simulink model "rlObstacleAvoidance"  (R2019b)
settings: Solver=ode23t  StartTime=0.0  StopTime=inf  RelTol=1e-3
InitFcn:
  | close all;
  | clear showPath;
  | lidarNoiseSeeds = randi(intmax,size(scanAngles));
model workspace (MAT data in the model file):
  mapForSim.obsMap = [0 0 0 0 0 0 0 0 0 0 0 0 ... (25000 elements, 200x125)]
  mapForSim.scaleFactor = 25
  mapForSim.simMap = robotics.BinaryOccupancyGrid
  mapForSim.simMap.Grid = [1 1 1 1 1 1 1 1 1 1 1 1 ... (25000 elements, 200x125)]
  mapForSim.simMap.LayerName = "binaryLayer"
  mapForSim.simMap.Index = matlabshared.autonomous.internal.CircularBufferIndex
  mapForSim.simMap.Index.Head = [1 1]
  mapForSim.simMap.Index.Size = [200 125]
  mapForSim.simMap.Index.NewRegions = [0 0 0 0]
  mapForSim.simMap.Index.DropEntireMap = 0
  mapForSim.simMap.Index.DropTwoRegions = [0 0]
  mapForSim.simMap.Buffer = matlabshared.autonomous.internal.CircularBuffer
  mapForSim.simMap.Buffer.ConstVal = 0
  mapForSim.simMap.Buffer.DataType = 'logical'
  mapForSim.simMap.Buffer.Index = matlabshared.autonomous.internal.CircularBufferIndex
  mapForSim.simMap.Buffer.Index.Head = [1 1]
  mapForSim.simMap.Buffer.Index.Size = [200 125]
  mapForSim.simMap.Buffer.Index.NewRegions = [0 0 0 0]
  mapForSim.simMap.Buffer.Index.DropEntireMap = 0
  mapForSim.simMap.Buffer.Index.DropTwoRegions = [0 0]
  mapForSim.simMap.Buffer.Buffer = [1 1 1 1 1 1 1 1 1 1 1 1 ... (25000 elements, 200x125)]
  mapForSim.simMap.DefaultValueInternal = 0
  mapForSim.simMap.HasParent = 0
  mapForSim.simMap.Resolution = 25
  mapForSim.simMap.GridSize = [200 125]
  mapForSim.simMap.GridOriginInLocal = [0 0]
  mapForSim.simMap.LocalOriginInWorld = [0 0]
  mapForSim.simMap.Width = 5
  mapForSim.simMap.Height = 8
  mapForSim.simMap.LocalOriginInWorldInternal = [0 0]
  occGrid = robotics.BinaryOccupancyGrid
  occGrid.Grid = [1 1 1 1 1 1 1 1 1 1 1 1 ... (25000 elements, 200x125)]
  occGrid.LayerName = "binaryLayer"
  occGrid.Index = matlabshared.autonomous.internal.CircularBufferIndex
  occGrid.Index.Head = [1 1]
  occGrid.Index.Size = [200 125]
  occGrid.Index.NewRegions = [0 0 0 0]
  occGrid.Index.DropEntireMap = 0
  occGrid.Index.DropTwoRegions = [0 0]
  occGrid.Buffer = matlabshared.autonomous.internal.CircularBuffer
  occGrid.Buffer.ConstVal = 0
  occGrid.Buffer.DataType = 'logical'
  occGrid.Buffer.Index = matlabshared.autonomous.internal.CircularBufferIndex
  occGrid.Buffer.Index.Head = [1 1]
  occGrid.Buffer.Index.Size = [200 125]
  occGrid.Buffer.Index.NewRegions = [0 0 0 0]
  occGrid.Buffer.Index.DropEntireMap = 0
  occGrid.Buffer.Index.DropTwoRegions = [0 0]
  occGrid.Buffer.Buffer = [1 1 1 1 1 1 1 1 1 1 1 1 ... (25000 elements, 200x125)]
  occGrid.DefaultValueInternal = 0
  occGrid.HasParent = 0
  occGrid.Resolution = 25
  occGrid.GridSize = [200 125]
  occGrid.GridOriginInLocal = [0 0]
  occGrid.LocalOriginInWorld = [0 0]
  occGrid.Width = 5
  occGrid.Height = 8
  occGrid.LocalOriginInWorldInternal = [0 0]
undefined symbols (not defined in the file or in its folder): lidarNoiseVariance, maxAngSpeed, maxLinSpeed, maxRange, sampleTime
libraries: simulink x3, mobileRoboticsLib x3, rllib x1
settings Model: Creator=josea  LastModifiedBy=scastro
settings DataIOCC: ReturnWorkspaceOutputs=off
settings DebuggingCC: UnconnectedLineMsg=none  PregeneratedLibrarySubsystemCodeDiagnostic=none  ArithmeticOperatorsInVariantConditions=warning
settings SFSimCC: SimUseLocalCustomCode=off  CustomCodeUndefinedFunction=UseInterfaceOnly
settings RTWCC: RTWUseLocalCustomCode=off
settings DiagnosticsConfigSet: SimMechanicsRigidlyBoundBlock=none
settings ExplorerConfigSet: InternalSimMechanicsExplorerSettings="<ExplorerConfiguration><canonicalview>default</canonicalview><AnimationSetting><BasePlaybackSpeed>1.0</BasePlaybackSpeed><PlaybackSpeedFactor>1.0</PlaybackSpeedFactor></AnimationSetting><TilePanel><TileInfo><Tiles Columns=\"2\" Count=\"3\" Rows=\"2\"><Column Weight=\"0.4996\"/><Column Weight=\"0.5004\"/><Row Weight=\"0.4995\"/><Row Weight=\"0.5005\"/><Tile Height=\"1\" Width=\"2\" X=\"0\" Y=\"0\"/><Tile Height=\"1\" Width=\"1\" X=\"0\" Y=\"1\"/><Tile Height=\"1\" Width=\"1\" X=\"1\" Y=\"1\"/></Tiles></TileInfo><SceneInfo><SceneViewer><BGColor><R>0.60000002384185791</R><G>0.60000002384185791</G><B>0.60000002384185791</B></BGColor><Camera><DoPerspective>off</DoPerspective><Position><X>3.21513503845026616</X><Y>-4.39133612297629217</Y><Z>3.60331941083972662</Z></Position><Center><X>0.446473736246977004</X><Y>-0.407537419322758776</Y><Z>0.493999065547941429</Z></Center><Up><X>-0.250055633923735143</X><Y>0.481736888045999345</Y><Z>0.839881986137787973</Z></Up><ViewLimDist>1</ViewLimDist><YLim>3.04422703072066758</YLim><XLim>7.99109595564175201</XLim></Camera></SceneViewer><SceneViewer><BGColor><R>0.60000002384185791</R><G>0.60000002384185791</G><B>0.60000002384185791</B></BGColor><Camera><DoPerspective>on</DoPerspective><Position><X>-0.900230893541791977</X><Y>-0.0744300644421216767</Y><Z>0.454136559277898921</Z></Position><Center><X>-1.83076580855623683</X><Y>-0.205300204269928455</Y><Z>0.112116415952230264</Z></Center><Up><X>-0.338687011010687988</X><Y>-0.047632835451577496</Y><Z>0.939692620785908428</Z></Up><ViewLimDist>1</ViewLimDist><YLim>0.466307658154998583</YLim><XLim>0.604541153655492214</XLim></Camera></SceneViewer><SceneViewer><BGColor><R>0.60000002384185791</R><G>0.60000002384185791</G><B>0.60000002384185791</B></BGColor><Camera><DoPerspective>off</DoPerspective><Position><X>-0.126032215770511102</X><Y>-0.027243386375953943</Y><Z>6.53261199512664703</Z></Position><Center><X>-0.126032215770511102</X><Y>-0.027243386375953943</Y><Z>0.127156752764657099</Z></Center><Up><X>0</X><Y>1</Y><Z>-0</Z></Up><ViewLimDist>1</ViewLimDist><YLim>4.0594907565083922</YLim><XLim>5.27894252526190133</XLim></Camera></SceneViewer></SceneInfo></TilePanel><MechEditorPanel><Cameras><Camera><Id>Camera1</Id><Value><Name>RobotView</Name><NativeCamera><PositionTrackingFeature>Obstacle_Environment.Robot.Body.RobotCamera.F</PositionTrackingFeature><CenterTrackingFeature>Obstacle_Environment.Robot.Body.RobotCamera.F</CenterTrackingFeature><UpVectorTrackingFeature>Obstacle_Environment.Robot.Body.RobotCamera.F</UpVectorTrackingFeature><CenterTrackingOrigin>off</CenterTrackingOrigin><CenterTrackingDirection>+X</CenterTrackingDirection><UpVectorTrackingDirection>+Z</UpVectorTrackingDirection></NativeCamera></Value></Camera></Cameras><GfxPanelCameraMap><MapElement CameraMLId=\"Camera1\" GfxPanelIndex=\"1\"/></GfxPanelCameraMap><VideoCreator><PlaybackSpeedRatio>1.0</PlaybackSpeedRatio><FrameRate>30</FrameRate><VideoFormat>Motion JPEG AVI</VideoFormat><FrameSize>auto</FrameSize></VideoCreator></MechEditorPanel></ExplorerConfiguration>"

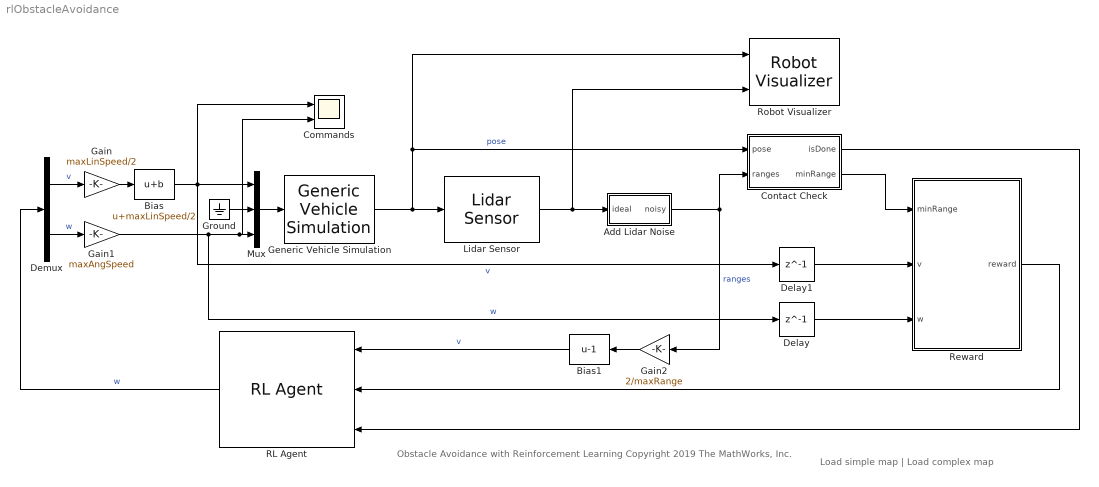
== system rlObstacleAvoidance ==
  note: Obstacle Avoidance with Reinforcement Learning
      | Copyright 2019 The MathWorks, Inc.
  note: Load simple map | Load complex map
  Add Lidar Noise : Subsystem
  Bias : Bias  Bias=maxLinSpeed/2
  Bias1 : Bias  Bias=-1
  Commands : Scope  NumInputPorts=2
  Contact Check : Subsystem
  Delay : Delay  DelayLength=1
  Delay1 : Delay  DelayLength=1
  Demux : Demux  Outputs=2
  Gain : Gain  Gain=maxLinSpeed/2
  Gain1 : Gain  Gain=maxAngSpeed
  Gain2 : Gain  Gain=2/maxRange
  Generic Vehicle Simulation : mobileRoboticsLib/Utilities/Generic Vehicle Simulation  initX=initX  initY=initY  initAngle=initTheta  Ts=sampleTime
      settings: SourceProductName=Mobile Robotics Simulation Library
  Ground : Ground
  Lidar Sensor : mobileRoboticsLib/Environments/Lidar Sensor  mapName=map  sensorOffset=[ 0 0 ]  scanAngles=scanAngles  maxRange=maxRange
      settings: SourceProductName=Ground Vehicles Library
  Mux : Mux  Inputs=3
  RL Agent : rllib/RL Agent  Agent=agent  ProvideReward=on  ProvideIsDone=on  ProvideCumRwd=off  TreatAsDirectFeedthrough=on  CollectLoggedSignals=on  CollectModelStates=on
      settings: SourceProductName=Reinforcement Learning Toolbox
  Reward : Subsystem
  Robot Visualizer : mobileRoboticsLib/Environments/Robot Visualizer  Priority=99  robotRadius=robotRadius  mapName=map  showTrajectory=on  hasWaypoints=off  hasLidar=on  sensorOffset=[ 0 0 ]  scanAngles=scanAngles  hasObjDetector=off  objDetectorOffset=[ 0, 0 ]  objDetectorAngle=0  objDetectorFOV=pi/4  objDetectorMaxRange=5  objectColors=[ 1, 0, 0; 0, 1, 0; 0, 0, 1 ]  objectMarkers='s'
      settings: SourceProductName=Ground Vehicles Library
  wires:
  Reward/1(reward) -> RL Agent/2
  Demux/2 -> Gain1/1  "w"
  Demux/1 -> Gain/1  "v"
  Mux/1 -> Generic Vehicle Simulation/1
  Generic Vehicle Simulation/1 -> Lidar Sensor/1, Robot Visualizer/1, Contact Check/1(pose)  "pose"
  Ground/1 -> Mux/2
  RL Agent/1 -> Demux/1  "w"
  Delay/1 -> Reward/3(w)
  Contact Check/2(minRange) -> Reward/1(minRange)
  Gain/1 -> Bias/1
  Bias/1 -> Mux/1, Delay1/1, Commands/1  "v"
  Gain1/1 -> Mux/3, Commands/2, Delay/1  "w"
  Delay1/1 -> Reward/2(v)
  Contact Check/1(isDone) -> RL Agent/3
  Add Lidar Noise/1(noisy) -> Gain2/1, Contact Check/2(ranges)  "ranges"
  Gain2/1 -> Bias1/1
  Bias1/1 -> RL Agent/1  "v"
  Lidar Sensor/1 -> Robot Visualizer/2, Add Lidar Noise/1(ideal)

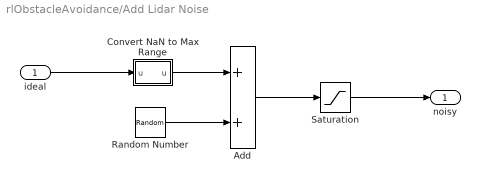
== system rlObstacleAvoidance/Add Lidar Noise ==
  ideal : Inport
  Add : Sum
  Convert NaN to Max Range : MATLAB Function  TreatAsAtomicUnit=on
  Random Number : RandomNumber  Variance=lidarNoiseVariance  Seed=lidarNoiseSeeds  SampleTime=sampleTime
  Saturation : Saturate  UpperLimit=inf  LowerLimit=0
  noisy : Outport
  wires:
  ideal/1 -> Convert NaN to Max Range/1("u ")
  Random Number/1 -> Add/2
  Add/1 -> Saturation/1
  Saturation/1 -> noisy/1
  Convert NaN to Max Range/1(u) -> Add/1

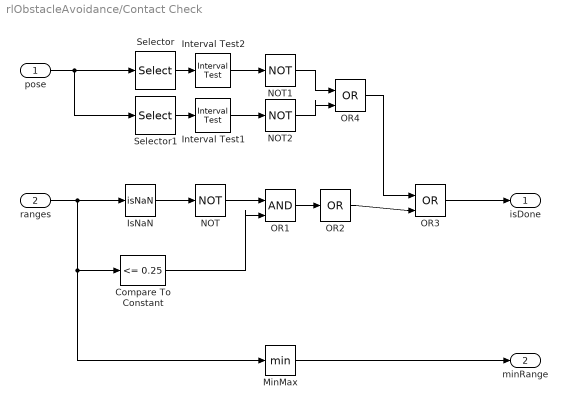
== system rlObstacleAvoidance/Contact Check ==
  pose : Inport
  ranges : Inport  Port=2
  Compare To Constant : simulink/Logic and Bit Operations/Compare To Constant  relop=<=  const=0.25  OutDataTypeStr=boolean
  Interval Test1 : simulink/Logic and Bit Operations/Interval Test  IntervalClosedRight=on  uplimit=13  IntervalClosedLeft=on  lowlimit=0  OutDataTypeStr=boolean
  Interval Test2 : simulink/Logic and Bit Operations/Interval Test  IntervalClosedRight=on  uplimit=13  IntervalClosedLeft=on  lowlimit=0  OutDataTypeStr=boolean
  IsNaN : RelationalOperator  Operator=isNaN  OutDataTypeStr=boolean  RndMeth=Simplest
  MinMax : MinMax
  NOT : Logic  Operator=NOT  IconShape=distinctive  AllPortsSameDT=off  OutDataTypeStr=boolean
  NOT1 : Logic  Operator=NOT  IconShape=distinctive  AllPortsSameDT=off  OutDataTypeStr=boolean
  NOT2 : Logic  Operator=NOT  IconShape=distinctive  AllPortsSameDT=off  OutDataTypeStr=boolean
  OR1 : Logic  IconShape=distinctive  AllPortsSameDT=off  OutDataTypeStr=boolean
  OR2 : Logic  Operator=OR  Inputs=1  IconShape=distinctive  AllPortsSameDT=off  OutDataTypeStr=boolean
  OR3 : Logic  Operator=OR  IconShape=distinctive  AllPortsSameDT=off  OutDataTypeStr=boolean
  OR4 : Logic  Operator=OR  IconShape=distinctive  AllPortsSameDT=off  OutDataTypeStr=boolean
  Selector : Selector  InputPortWidth=3  IndexOptions=Index vector (dialog)  Indices=1  OutputSizes=1
  Selector1 : Selector  InputPortWidth=3  IndexOptions=Index vector (dialog)  Indices=2  OutputSizes=1
  isDone : Outport  VectorParamsAs1DForOutWhenUnconnected=off
  minRange : Outport  Port=2  VectorParamsAs1DForOutWhenUnconnected=off
  wires:
  OR1/1 -> OR2/1
  Compare To Constant/1 -> OR1/2
  NOT/1 -> OR1/1
  ranges/1 -> MinMax/1, Compare To Constant/1, IsNaN/1
  IsNaN/1 -> NOT/1
  MinMax/1 -> minRange/1
  OR3/1 -> isDone/1
  pose/1 -> Selector/1, Selector1/1
  Selector/1 -> Interval Test2/1
  Selector1/1 -> Interval Test1/1
  OR2/1 -> OR3/2
  NOT1/1 -> OR4/1
  Interval Test1/1 -> NOT2/1
  OR4/1 -> OR3/1
  Interval Test2/1 -> NOT1/1
  NOT2/1 -> OR4/2

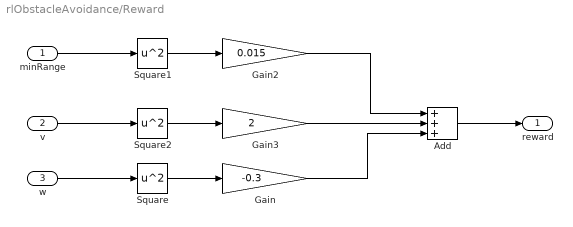
== system rlObstacleAvoidance/Reward ==
  minRange : Inport
  v : Inport  Port=2
  w : Inport  Port=3
  Add : Sum  Inputs=+++
  Gain : Gain  Gain=-0.3
  Gain2 : Gain  Gain=0.015
  Gain3 : Gain  Gain=2
  Square : Math  Operator=square  SaturateOnIntegerOverflow=on
  Square1 : Math  Operator=square  SaturateOnIntegerOverflow=on
  Square2 : Math  Operator=square  SaturateOnIntegerOverflow=on
  reward : Outport  VectorParamsAs1DForOutWhenUnconnected=off
  wires:
  Square/1 -> Gain/1
  w/1 -> Square/1
  Gain/1 -> Add/3
  minRange/1 -> Square1/1
  Gain2/1 -> Add/1
  Square1/1 -> Gain2/1
  v/1 -> Square2/1
  Square2/1 -> Gain3/1
  Gain3/1 -> Add/2
  Add/1 -> reward/1

== matlab function rlObstacleAvoidance/Add Lidar Noise/Convert NaN to Max Range ==
  data: u input; u output; maxRange parameter
function u = removeNans(u,maxRange)

u(isnan(u)) = maxRange;
